simulink model "msfcndemo_vsfunc"  (Simulink 7.6)
settings: Solver=ode45  StartTime=0.0  StopTime=50  RelTol=1e-3
settings Model: Creator=The MathWorks Inc.  ExtModeTrigMode=oneshot  ExtModeArmWhenConnect=off  ExtModeAutoUpdateStatusClock=off
settings DataIOCC: LimitDataPoints=off  SaveFormat=StructureWithTime  SaveState=on  OutputSaveName=yout1
settings OptimizationCC: BlockReduction=off  BooleanDataType=off  InlineInvariantSignals=on  InitFltsAndDblsToZero=on
settings DebuggingCC: SaveWithParameterizedLinksMsg=none  SignalResolutionControl=TryResolveAllWithWarning  SolverPrmCheckMsg=none  MultiTaskDSMMsg=warning  MultiTaskCondExecSysMsg=none
settings HardwareCC: TargetUnknown=on
settings RTWCC: IncludeERTFirstTime=on
settings GRTTargetCC: TargetFcnLib=ansi_tfl_tmw.mat

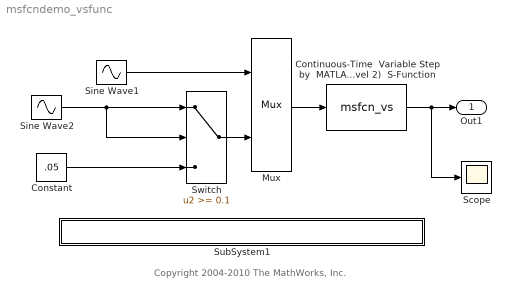
== system msfcndemo_vsfunc ==
  note: Copyright 2004-2010 The MathWorks, Inc.
  Constant : Constant  Value=.05
  Continuous-Time  Variable Step by  MATLAB file (level 2)  S-Function : M-S-Function  FunctionName=msfcn_vs
      mask Display: disp('dt           = u(2)\ny(t + dt) = u(t)')
  Mux : Mux  Inputs=2
  Scope : Scope
      settings: TimeRange=50  YMin=-1  YMax=1  SaveName=scopeout1
  Sine Wave1 : Sin  Frequency=2*pi  SampleTime=0
  Sine Wave2 : Sin  Amplitude=2  Frequency=2*pi  SampleTime=0
  SubSystem1 : Subsystem  mask{filename=msfcn_vs.m}
      mask init:
      | x=sfundemo_maskdisp;
      settings: AttributesFormatString=\n  OpenFcn=sfundemo_openfcn
      mask Display: disp(['MATLAB file: ' x]);
  Switch : Switch  Threshold=0.1  SaturateOnIntegerOverflow=on  InputSameDT=on
  Out1 : Outport  InitialOutput=0
  wires:
  Constant/1 -> Switch/3
  Mux/1 -> Continuous-Time  Variable Step by  MATLAB file (level 2)  S-Function/1
  Sine Wave2/1 -> Switch/1, Switch/2
  Continuous-Time  Variable Step by  MATLAB file (level 2)  S-Function/1 -> Out1/1, Scope/1
  Sine Wave1/1 -> Mux/1
  Switch/1 -> Mux/2

== system msfcndemo_vsfunc/SubSystem1 ==
